simulink model "Simulink_Program"  (R2023b)
settings: Solver=VariableStepAuto  StartTime=0.0  StopTime=1  RelTol=1e-3
undefined symbols (not defined in the file or in its folder): battery_builder_rtmsupport, gcbh, Ns_Module, NumModules
libraries: nesl_utility x52, BatteryPack_105s34p_Library_lib x36, fl_lib x17, ee_lib x7
(part 1 of 5)
settings Model: Creator=romul  LastModifiedBy=OWNER

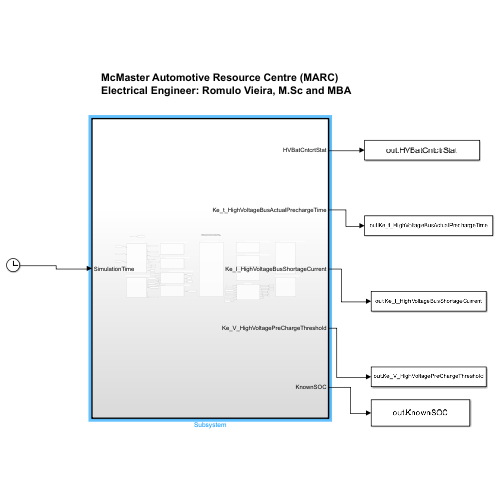
[thumbnail: Simulink's stored preview of the top-level diagram]
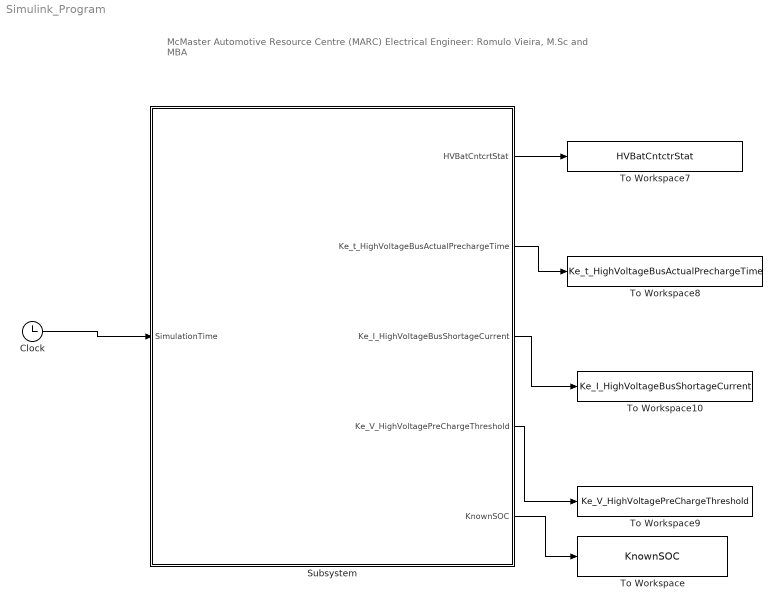
== system Simulink_Program ==
  note: McMaster Automotive Resource Centre (MARC)
      | Electrical Engineer: Romulo Vieira, M.Sc and MBA
  Clock : Clock
  Subsystem : Subsystem  TreatAsAtomicUnit=on
  To Workspace : ToWorkspace  VariableName=KnownSOC  SaveFormat=Timeseries  SampleTime=-1
  To Workspace10 : ToWorkspace  VariableName=Ke_I_HighVoltageBusShortageCurrent  SampleTime=-1
  To Workspace7 : ToWorkspace  VariableName=HVBatCntctrStat  SampleTime=-1
  To Workspace8 : ToWorkspace  VariableName=Ke_t_HighVoltageBusActualPrechargeTime  SampleTime=-1
  To Workspace9 : ToWorkspace  VariableName=Ke_V_HighVoltagePreChargeThreshold  SampleTime=-1
  wires:
  Subsystem/1(HVBatCntcrtStat) -> To Workspace7/1
  Subsystem/2(Ke_t_HighVoltageBusActualPrechargeTime) -> To Workspace8/1
  Subsystem/3(Ke_I_HighVoltageBusShortageCurrent) -> To Workspace10/1
  Clock/1 -> Subsystem/1(SimulationTime)
  Subsystem/4(Ke_V_HighVoltagePreChargeThreshold) -> To Workspace9/1
  Subsystem/5(KnownSOC) -> To Workspace/1

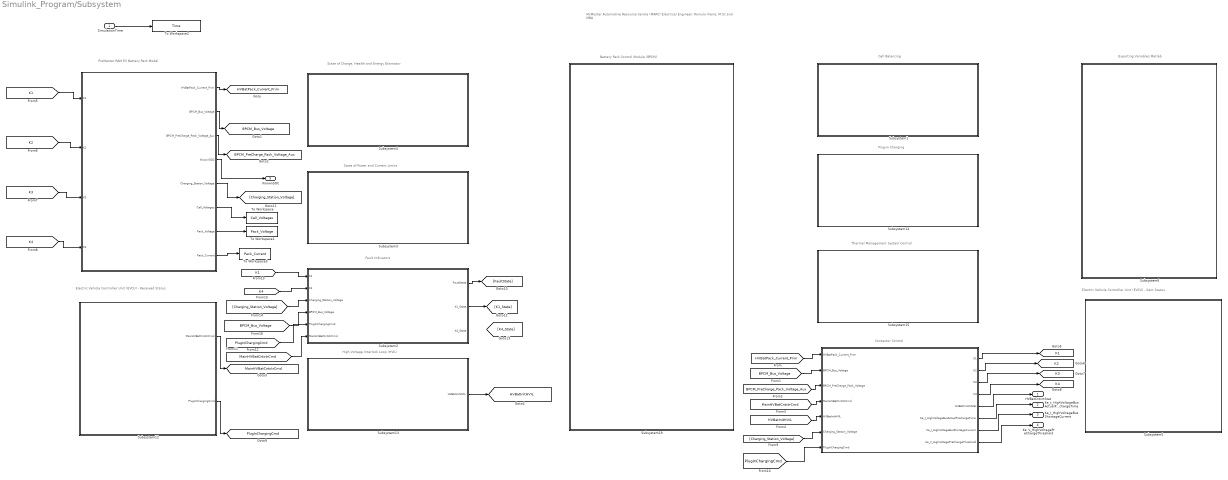
== system Simulink_Program/Subsystem ==
  note: McMaster Automotive Resource Centre (MARC)
      | Electrical Engineer: Romulo Vieira, M.Sc and MBA
  note: ProMaster RAM EV Battery Pack Model
  note: Contactor Control
  note: Battery Pack Control Module (BPCM)
  note: Thermal Management System Control
  note: Plug-In Charging
  note: Cell Balancing
  note: High Voltage Interlock Loop (HVIL)
  note: Fault Indicators
  note: State of Power and Current Limits
  note: State of Charge, Health and Energy Estimator
  note: Electric Vehicle Controller Unit (EVCU) - Received Status
  note: Electric Vehicle Controller Unit (EVCU) - Sent Status
  note: Exporting Variables Matlab
  SimulationTime : Inport
  " " : Subsystem  TreatAsAtomicUnit=on
  "  " : Subsystem  TreatAsAtomicUnit=on  SystemSampleTime=0.001
  Subsystem1 : Subsystem
  Subsystem12 : Subsystem
  Subsystem13 : Subsystem
  Subsystem14 : Subsystem
  Subsystem15 : Subsystem
  Subsystem19 : Subsystem
  Subsystem2 : Subsystem
  Subsystem3 : Subsystem
  Subsystem4 : Subsystem
  Subsystem5 : Subsystem
  Subsystem6 : Subsystem
  To Workspace : ToWorkspace  VariableName=Cell_Voltages  SaveFormat=Timeseries  SampleTime=-1
  To Workspace1 : ToWorkspace  VariableName=Pack_Voltage  SaveFormat=Timeseries  SampleTime=-1
  To Workspace2 : ToWorkspace  VariableName=Time  SampleTime=0.001
  To Workspace3 : ToWorkspace  VariableName=Pack_Current  SaveFormat=Timeseries  SampleTime=-1
  HVBatCntcrtStat : Outport
  Ke_t_HighVoltageBusActualPrechargeTime : Outport  Port=2
  Ke_I_HighVoltageBusShortageCurrent : Outport  Port=3
  Ke_V_HighVoltagePreChargeThreshold : Outport  Port=4
  KnownSOC : Outport  Port=5
  tag scope: BPCM_Bus_Voltage=global, BPCM_PreCharge_Pack_Voltage_Aux=global, HVBatInitHVIL=global, HVBatPack_Current_Prim=global, K1=global, K2=global, K3=global, K4=global, MainHVBatCntctrCmd=global, PlugInChargingCmd=global
  wires:
  "  "/5(HVBatCntctrStat) -> HVBatCntcrtStat/1
  "  "/6(Ke_t_HighVoltageBusActualPrechargeTime) -> Ke_t_HighVoltageBusActualPrechargeTime/1
  "  "/7(Ke_I_HighVoltageBusShortageCurrent) -> Ke_I_HighVoltageBusShortageCurrent/1
  "  "/8(Ke_V_HighVoltagePreChargeThreshold) -> Ke_V_HighVoltagePreChargeThreshold/1
  SimulationTime/1 -> To Workspace2/1
  " "/1(HVBatPack_Current_Prim) -> [HVBatPack_Current_Prim]
  " "/2(BPCM_Bus_Voltage) -> [BPCM_Bus_Voltage]
  " "/3(BPCM_PreCharge_Pack_Voltage_Aux) -> [BPCM_PreCharge_Pack_Voltage_Aux]
  [HVBatPack_Current_Prim] -> "  "/1(HVBatPack_Current_Prim)
  [BPCM_Bus_Voltage] -> "  "/2(BPCM_Bus_Voltage)
  [BPCM_PreCharge_Pack_Voltage_Aux] -> "  "/3(BPCM_PreCharge_Pack_Voltage)
  Subsystem12/1(" MainHVBatCntctrCmd      ") -> [MainHVBatCntctrCmd]
  [MainHVBatCntctrCmd] -> "  "/4(MainHVBatCntctrCmd)
  Subsystem13/1("HVBatInitHVIL   ") -> [HVBatInitHVIL]
  [HVBatInitHVIL] -> "  "/5(HVBatInitHVIL)
  "  "/3(K3) -> [K3]
  "  "/4(K4) -> [K4]
  "  "/1(K1) -> [K1]
  "  "/2(K2) -> [K2]
  [K1] -> " "/1(K1)
  [K2] -> " "/2(K2)
  [K3] -> " "/3(K3)
  [K4] -> " "/4(K4)
  " "/4(KnownSOC) -> KnownSOC/1
  " "/5(Charging_Station_Voltage) -> [Charging_Station_Voltage]
  [Charging_Station_Voltage] -> "  "/6(Charging_Station_Voltage)
  " "/6(Cell_Voltages) -> To Workspace/1
  " "/7(Pack_Voltage) -> To Workspace1/1
  " "/8(Pack_Current) -> To Workspace3/1
  [PlugInChargingCmd] -> "  "/7(PlugInChargingCmd)
  Subsystem12/2(" PlugInChargingCmd      ") -> [PlugInChargingCmd]
  [K1] -> Subsystem2/1(K1)
  [BPCM_Bus_Voltage] -> Subsystem2/4(BPCM_Bus_Voltage)
  [K4] -> Subsystem2/2(K4)
  [Charging_Station_Voltage] -> Subsystem2/3(Charging_Station_Voltage)
  [PlugInChargingCmd] -> Subsystem2/5(PlugInChargingCmd)
  [MainHVBatCntctrCmd] -> Subsystem2/6(MainHVBatCntctrCmd)
  Subsystem2/1(FaultState) -> [FaultState]
  Subsystem2/2(K1_State) -> [K1_State]

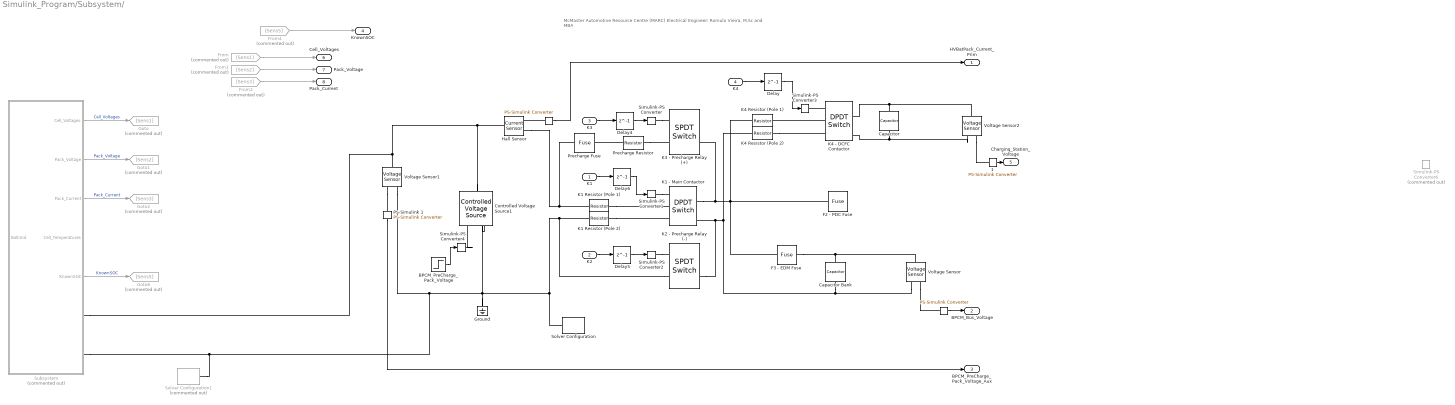
== system Simulink_Program/Subsystem/  ==
  note: McMaster Automotive Resource Centre (MARC)
      | Electrical Engineer: Romulo Vieira, M.Sc and MBA
  K1 : Inport
  K2 : Inport  Port=2
  K3 : Inport  Port=3
  K4 : Inport  Port=4
  "   " : nesl_utility/PS-Simulink Converter  PhysicalDomain=network_engine_domain  SubClassName=ps_output  LeftPortType=input  RightPortType=output  PseudoPeriodic=off  Frequencies=[]  VectorFormat=inherit  Unit=inherit  AffineConversion=off
  " " : nesl_utility/PS-Simulink Converter  PhysicalDomain=network_engine_domain  SubClassName=ps_output  LeftPortType=input  RightPortType=output  PseudoPeriodic=off  Frequencies=[]  VectorFormat=inherit  Unit=inherit  AffineConversion=off
  " 1" : nesl_utility/PS-Simulink Converter  PhysicalDomain=network_engine_domain  SubClassName=ps_output  LeftPortType=input  RightPortType=output  PseudoPeriodic=off  Frequencies=[]  VectorFormat=inherit  Unit=inherit  AffineConversion=off
  BPCM_PreCharge_Pack_Voltage : Step  Time=0  After=450  SampleTime=0.001
  Capacitor : fl_lib/Electrical/Electrical Elements/Capacitor  c=750e-6 F  r=1e-6 Ohm  g=0 1/Ohm  i_specify=off  i_priority=None  i=0 A  i_nominal_specify=off  i_nominal_unit=A  i_nominal_value=1  v_specify=off  v_priority=None  v=0 V  v_nominal_specify=off  v_nominal_unit=V  v_nominal_value=1  vc_specify=off  vc_priority=High  vc=0 V  vc_nominal_specify=off  vc_nominal_unit=V  vc_nominal_value=1
  Capacitor Bank : fl_lib/Electrical/Electrical Elements/Capacitor  c=750e-6 F  r=1e-6 Ohm  g=0 1/Ohm  i_specify=off  i_priority=None  i=0 A  i_nominal_specify=off  i_nominal_unit=A  i_nominal_value=1  v_specify=off  v_priority=None  v=0 V  v_nominal_specify=off  v_nominal_unit=V  v_nominal_value=1  vc_specify=on  vc_priority=High  vc=0 V  vc_nominal_specify=off  vc_nominal_unit=V  vc_nominal_value=1
  Controlled Voltage Source1 : fl_lib/Electrical/Electrical Sources/Controlled Voltage Source
  Delay{,4..6} (4 alike) : Delay  DelayLength=1
  F2 - PDC Fuse : ee_lib/Switches & Breakers/Fuse  prm=1  I_rated=125 A  melt_margin=1  T_fuse=0 s  I2t=1 A^2*s  I_vec=[1.9, 2, 2.5, 30] A  t_vec=[10000, 1, .3, .001] s  R_closed=0.01 Ohm  G_open=1e-8 1/Ohm  exposemeasurement=ee.enum.exposemeasurement.hidden
      settings: InternalSimscapePortConfiguration="{\"Bottom\":[],\"Left\":[{\"id\":\"p\",\"label\":\"\",\"type\":\"foundation.electrical.electrical\"}],\"Right\":[{\"id\":\"n\",\"label\":\"\",\"type\":\"foundation.electrical.electrical\"}],\"Top\":[]}"
  F3 - EDM Fuse : ee_lib/Switches & Breakers/Fuse  prm=1  I_rated=600 A  melt_margin=1  T_fuse=0 s  I2t=1 A^2*s  I_vec=[1.9, 2, 2.5, 30] A  t_vec=[10000, 1, .3, .001] s  R_closed=0.01 Ohm  G_open=1e-8 1/Ohm  exposemeasurement=ee.enum.exposemeasurement.hidden
      settings: InternalSimscapePortConfiguration="{\"Bottom\":[],\"Left\":[{\"id\":\"p\",\"label\":\"\",\"type\":\"foundation.electrical.electrical\"}],\"Right\":[{\"id\":\"n\",\"label\":\"\",\"type\":\"foundation.electrical.electrical\"}],\"Top\":[]}"
  From : From  Commented=on  GotoTag=Sens1
  From1 : From  Commented=on  GotoTag=Sens2
  From2 : From  Commented=on  GotoTag=Sens3
  From4 : From  Commented=on  GotoTag=Sens5
  Goto : Goto  Commented=on  GotoTag=Sens1
  Goto1 : Goto  Commented=on  GotoTag=Sens2
  Goto2 : Goto  Commented=on  GotoTag=Sens3
  Goto6 : Goto  Commented=on  GotoTag=Sens5
  Ground : fl_lib/Electrical/Electrical Elements/Electrical Reference
  Hall Sensor : fl_lib/Electrical/Electrical Sensors/Current Sensor
  K1 - Main Contactor : ee_lib/Switches & Breakers/DPDT Switch  R_closed=0.01 Ohm  G_open=1e-6 S  Threshold=0.5 V  Width=0 V  model_dynamics=0  t_on=1e-3 s  t_off=1e-3 s  initial_vT=0 V
      settings: InternalSimscapePortConfiguration="{\"Bottom\":[],\"Left\":[{\"id\":\"vT\",\"label\":\"vT\",\"type\":\"input\"},{\"id\":\"p1\",\"label\":\"\",\"type\":\"foundation.electrical.electrical\"},{\"id\":\"p2\",\"label\":\"\",\"type\":\"foundation.electrical.electrical\"}],\"Right\":[{\"id\":\"n11\",\"label\":\"\",\"type\":\"foundation.electrical.electrical\"},{\"id\":\"n12\",\"label\":\"\",\"type\":\"foundation.electrical.electrical\"},{\"id\":\"n21\",\"label\":\"\",\"type\":\"foundation.electrical.electrical\"},{\"id\":\"n22\",\"label\":\"\",\"type\":\"foundation.electrical.electrical\"}],\"Top\":[]}"
  K1 Resistor (Pole 1) : fl_lib/Electrical/Electrical Elements/Resistor  R=0.0003 Ohm  i_specify=off  i_priority=None  i=0 A  i_nominal_specify=off  i_nominal_unit=A  i_nominal_value=1  v_specify=off  v_priority=None  v=0 V  v_nominal_specify=off  v_nominal_unit=V  v_nominal_value=1
  K1 Resistor (Pole 2) : fl_lib/Electrical/Electrical Elements/Resistor  R=0.0003 Ohm  i_specify=off  i_priority=None  i=0 A  i_nominal_specify=off  i_nominal_unit=A  i_nominal_value=1  v_specify=off  v_priority=None  v=0 V  v_nominal_specify=off  v_nominal_unit=V  v_nominal_value=1
  K2 - Precharge Relay (-) : ee_lib/Switches & Breakers/SPDT Switch  R_closed=0.01 Ohm  G_open=1e-6 S  Threshold=0.5 V  Width=0 V  model_dynamics=0  t_on=1e-3 s  t_off=1e-3 s  initial_vT=0 V
  K3 - Precharge Relay (+) : ee_lib/Switches & Breakers/SPDT Switch  R_closed=0.01 Ohm  G_open=1e-6 S  Threshold=0.5 V  Width=0 V  model_dynamics=0  t_on=1e-3 s  t_off=1e-3 s  initial_vT=0 V
  K4 - DCFC Contactor : ee_lib/Switches & Breakers/DPDT Switch  R_closed=0.01 Ohm  G_open=1e-6 S  Threshold=0.5 V  Width=0 V  model_dynamics=0  t_on=1e-3 s  t_off=1e-3 s  initial_vT=0 V
      settings: InternalSimscapePortConfiguration="{\"Bottom\":[],\"Left\":[{\"id\":\"vT\",\"label\":\"vT\",\"type\":\"input\"},{\"id\":\"p1\",\"label\":\"\",\"type\":\"foundation.electrical.electrical\"},{\"id\":\"p2\",\"label\":\"\",\"type\":\"foundation.electrical.electrical\"}],\"Right\":[{\"id\":\"n11\",\"label\":\"\",\"type\":\"foundation.electrical.electrical\"},{\"id\":\"n12\",\"label\":\"\",\"type\":\"foundation.electrical.electrical\"},{\"id\":\"n21\",\"label\":\"\",\"type\":\"foundation.electrical.electrical\"},{\"id\":\"n22\",\"label\":\"\",\"type\":\"foundation.electrical.electrical\"}],\"Top\":[]}"
  K4 Resistor (Pole 1) : fl_lib/Electrical/Electrical Elements/Resistor  R=0.0003 Ohm  i_specify=off  i_priority=None  i=0 A  i_nominal_specify=off  i_nominal_unit=A  i_nominal_value=1  v_specify=off  v_priority=None  v=0 V  v_nominal_specify=off  v_nominal_unit=V  v_nominal_value=1
  K4 Resistor (Pole 2) : fl_lib/Electrical/Electrical Elements/Resistor  R=0.0003 Ohm  i_specify=off  i_priority=None  i=0 A  i_nominal_specify=off  i_nominal_unit=A  i_nominal_value=1  v_specify=off  v_priority=None  v=0 V  v_nominal_specify=off  v_nominal_unit=V  v_nominal_value=1
  PS-Simulink 1 : nesl_utility/PS-Simulink Converter  PhysicalDomain=network_engine_domain  SubClassName=ps_output  LeftPortType=input  RightPortType=output  PseudoPeriodic=off  Frequencies=[]  VectorFormat=inherit  Unit=inherit  AffineConversion=off
  Precharge Fuse : ee_lib/Switches & Breakers/Fuse  prm=1  I_rated=600 A  melt_margin=1  T_fuse=0 s  I2t=1 A^2*s  I_vec=[1.9, 2, 2.5, 30] A  t_vec=[10000, 1, .3, .001] s  R_closed=0.01 Ohm  G_open=1e-8 1/Ohm  exposemeasurement=ee.enum.exposemeasurement.hidden
      settings: InternalSimscapePortConfiguration="{\"Bottom\":[],\"Left\":[{\"id\":\"p\",\"label\":\"\",\"type\":\"foundation.electrical.electrical\"}],\"Right\":[{\"id\":\"n\",\"label\":\"\",\"type\":\"foundation.electrical.electrical\"}],\"Top\":[]}"
  Precharge Resistor : fl_lib/Electrical/Electrical Elements/Resistor  R=25 Ohm  i_specify=off  i_priority=None  i=0 A  i_nominal_specify=off  i_nominal_unit=A  i_nominal_value=1  v_specify=off  v_priority=None  v=0 V  v_nominal_specify=off  v_nominal_unit=V  v_nominal_value=1
  Simulink-PS Converter{,1..3} (4 alike) : nesl_utility/Simulink-PS Converter  PhysicalDomain=network_engine_domain  SubClassName=ps_input  LeftPortType=input  RightPortType=output  PseudoPeriodic=off  Frequencies=[]  NoiseDistribution=none  NoiseParameters=[]  Unit=1  AffineConversion=off  FilteringAndDerivatives=provide  SimscapeFilterOrder=1  InputFilterTimeConstant=0.001  UdotUserProvided=0
  Simulink-PS Converter4 : nesl_utility/Simulink-PS Converter  PhysicalDomain=network_engine_domain  SubClassName=ps_input  LeftPortType=input  RightPortType=output  PseudoPeriodic=off  Frequencies=[]  NoiseDistribution=none  NoiseParameters=[]  Unit=1  AffineConversion=off  FilteringAndDerivatives=filter  SimscapeFilterOrder=1  InputFilterTimeConstant=0.0000001  UdotUserProvided=0
  Simulink-PS Converter6 : nesl_utility/Simulink-PS Converter  Commented=on  PhysicalDomain=network_engine_domain  SubClassName=ps_input  LeftPortType=input  RightPortType=output  PseudoPeriodic=off  Frequencies=[]  NoiseDistribution=none  NoiseParameters=[]  Unit=1  AffineConversion=off  FilteringAndDerivatives=provide  SimscapeFilterOrder=1  InputFilterTimeConstant=0.001  UdotUserProvided=0
  Solver Configuration : nesl_utility/Solver Configuration  PhysicalDomain=network_engine_domain  SubClassName=solver  LeftPortType=input  RightPortType=generic  Tones=[]  Harmonics=[]  SimulateNoise=off  Profile=off  UseLocalSampling=off  EnableSwitchedLinearOptims=on  FrequencyDomain=off  UseCCode=off  RelTol=0.001  AbsTol=0.001  MinStep=1e-09  ToWorkspace=off  RevertToSquareIcSolve=off  NumHomotopyIterations=100  PhasorMode=off  PhasorModeNumHarmonics=1  ConsistencySolver=NEWTON_XTOL_AFTER_FTOL  IndexReductionMethod=DerivativeReplacement  DoDC=off  ResidualTolerance=1e-09  ConsistencyTolSource=GLOBAL  ConsistencyAbsTol=0.001  ConsistencyRelTol=0.001  ConsistencyTolFactor=0.001  UseLocalSolver=on  LocalSolverChoice=NE_BACKWARD_EULER_ADVANCER  ResolveIndetEquations=on  FunctionEvalNumThread=1  LocalSolverSampleTime=0.001  DoFixedCost=on  MaxNonlinIter=3  MaxModeIter=2  ComputeImpulses=off  ImpulseIterations=2  LinearAlgebra=auto  LinearAlgebraNumThread=0  EquationFormulation=NE_TIME_EF  DelaysMemoryBudget=1024  AutomaticFiltering=off  FilteringTimeConstant=0.001  PartitionStorageMethod=AS_NEEDED  PartitionMemoryBudget=1024  PartitionMethod=ROBUST  MultibodyUseLocalSolver=off  MultibodyLocalSolverChoice=ODE1  MultibodyLocalSolverSampleTime=0.001
  Solver Configuration1 : nesl_utility/Solver Configuration  Commented=on  PhysicalDomain=network_engine_domain  SubClassName=solver  LeftPortType=input  RightPortType=generic  Tones=[]  Harmonics=[]  SimulateNoise=off  Profile=off  UseLocalSampling=off  EnableSwitchedLinearOptims=on  FrequencyDomain=off  UseCCode=off  RelTol=0.001  AbsTol=0.001  MinStep=1e-09  ToWorkspace=off  RevertToSquareIcSolve=off  NumHomotopyIterations=100  PhasorMode=off  PhasorModeNumHarmonics=1  ConsistencySolver=NEWTON_XTOL_AFTER_FTOL  IndexReductionMethod=DerivativeReplacement  DoDC=off  ResidualTolerance=1e-09  ConsistencyTolSource=GLOBAL  ConsistencyAbsTol=0.001  ConsistencyRelTol=0.001  ConsistencyTolFactor=0.001  UseLocalSolver=on  LocalSolverChoice=NE_BACKWARD_EULER_ADVANCER  ResolveIndetEquations=on  FunctionEvalNumThread=1  LocalSolverSampleTime=0.001  DoFixedCost=on  MaxNonlinIter=3  MaxModeIter=2  ComputeImpulses=off  ImpulseIterations=2  LinearAlgebra=auto  LinearAlgebraNumThread=0  EquationFormulation=NE_TIME_EF  DelaysMemoryBudget=1024  AutomaticFiltering=off  FilteringTimeConstant=0.001  PartitionStorageMethod=AS_NEEDED  PartitionMemoryBudget=1024  PartitionMethod=ROBUST  MultibodyUseLocalSolver=off  MultibodyLocalSolverChoice=ODE1  MultibodyLocalSolverSampleTime=0.001
  Subsystem : Subsystem  Commented=on
      mask Display: image('saft-stellantis.jpg', [20, 45, 120, 70]);
  Voltage Sensor : fl_lib/Electrical/Electrical Sensors/Voltage Sensor
  Voltage Sensor1 : fl_lib/Electrical/Electrical Sensors/Voltage Sensor
  Voltage Sensor2 : fl_lib/Electrical/Electrical Sensors/Voltage Sensor
  HVBatPack_Current_Prim : Outport
  BPCM_Bus_Voltage : Outport  Port=2
  BPCM_PreCharge_Pack_Voltage_Aux : Outport  Port=3
  KnownSOC : Outport  Port=4  VectorParamsAs1DForOutWhenUnconnected=off  BusOutputAsStruct=on
  Charging_Station_Voltage : Outport  Port=5
  Cell_Voltages : Outport  Port=6
  Pack_Voltage : Outport  Port=7
  Pack_Current : Outport  Port=8
  wires:
  "   "/1 -> HVBatPack_Current_Prim/1
  K1/1 -> Delay6/1
  K2/1 -> Delay5/1
  BPCM_PreCharge_Pack_Voltage/1 -> Simulink-PS Converter4/1
  K3/1 -> Delay4/1
  Delay4/1 -> Simulink-PS Converter/1
  K4/1 -> Delay/1
  Delay5/1 -> Simulink-PS Converter2/1
  PS-Simulink 1/1 -> BPCM_PreCharge_Pack_Voltage_Aux/1
  " "/1 -> BPCM_Bus_Voltage/1
  Subsystem/1(Cell_Voltages) -> Goto/1  "Cell_Voltages"
  Subsystem/5(KnownSOC) -> Goto6/1  "KnownSOC"
  Subsystem/3(Pack_Current) -> Goto2/1  "Pack_Current"
  Subsystem/2(Pack_Voltage) -> Goto1/1  "Pack_Voltage"
  From1/1 -> Pack_Voltage/1
  From/1 -> Cell_Voltages/1
  From4/1 -> KnownSOC/1
  From2/1 -> Pack_Current/1
  " 1"/1 -> Charging_Station_Voltage/1
  Delay6/1 -> Simulink-PS Converter1/1
  Delay/1 -> Simulink-PS Converter3/1
  connections:
  K1 Resistor (Pole 2)/LConn1 -- K1 - Main Contactor/LConn3
  Capacitor Bank/LConn1 -- Voltage Sensor/LConn1 -- F3 - EDM Fuse/LConn1
  K2 - Precharge Relay (-)/RConn2 -- K1 - Main Contactor/RConn4 -- Voltage Sensor/RConn2 -- Capacitor Bank/RConn1 -- K4 Resistor (Pole 2)/RConn1
  Hall Sensor/RConn2 -- Precharge Fuse/LConn1 -- K1 Resistor (Pole 1)/RConn1
  K3 - Precharge Relay (+)/RConn2 -- K4 Resistor (Pole 1)/RConn1 -- F2 - PDC Fuse/RConn1 -- F3 - EDM Fuse/RConn1 -- K1 - Main Contactor/RConn2
  Precharge Resistor/LConn1 -- K3 - Precharge Relay (+)/LConn2
  Simulink-PS Converter2/RConn1 -- K2 - Precharge Relay (-)/LConn1
  Precharge Resistor/RConn1 -- Precharge Fuse/RConn1
  Simulink-PS Converter1/RConn1 -- K1 - Main Contactor/LConn1
  Controlled Voltage Source1/LConn1 -- Subsystem/RConn1 -- Voltage Sensor1/LConn1 -- Hall Sensor/LConn1
  Simulink-PS Converter/RConn1 -- K3 - Precharge Relay (+)/LConn1
  Voltage Sensor/RConn1 -- " "/LConn1
  K4 - DCFC Contactor/LConn1 -- Simulink-PS Converter3/RConn1
  "   "/LConn1 -- Hall Sensor/RConn1
  Simulink-PS Converter4/RConn1 -- Controlled Voltage Source1/RConn1
  Voltage Sensor1/RConn1 -- PS-Simulink 1/LConn1
  K1 Resistor (Pole 1)/LConn1 -- K1 - Main Contactor/LConn2
  Solver Configuration/RConn1 -- Solver Configuration1/RConn1 -- Subsystem/RConn2 -- Voltage Sensor1/RConn2 -- Ground/LConn1 -- Controlled Voltage Source1/RConn2 -- K2 - Precharge Relay (-)/LConn2 -- K1 Resistor (Pole 2)/RConn1
  K4 - DCFC Contactor/LConn2 -- K4 Resistor (Pole 1)/LConn1
  K4 Resistor (Pole 2)/LConn1 -- K4 - DCFC Contactor/LConn3
  Voltage Sensor2/LConn1 -- Capacitor/LConn1 -- K4 - DCFC Contactor/RConn2
  Voltage Sensor2/RConn2 -- K4 - DCFC Contactor/RConn4 -- Capacitor/RConn1
  Voltage Sensor2/RConn1 -- " 1"/LConn1

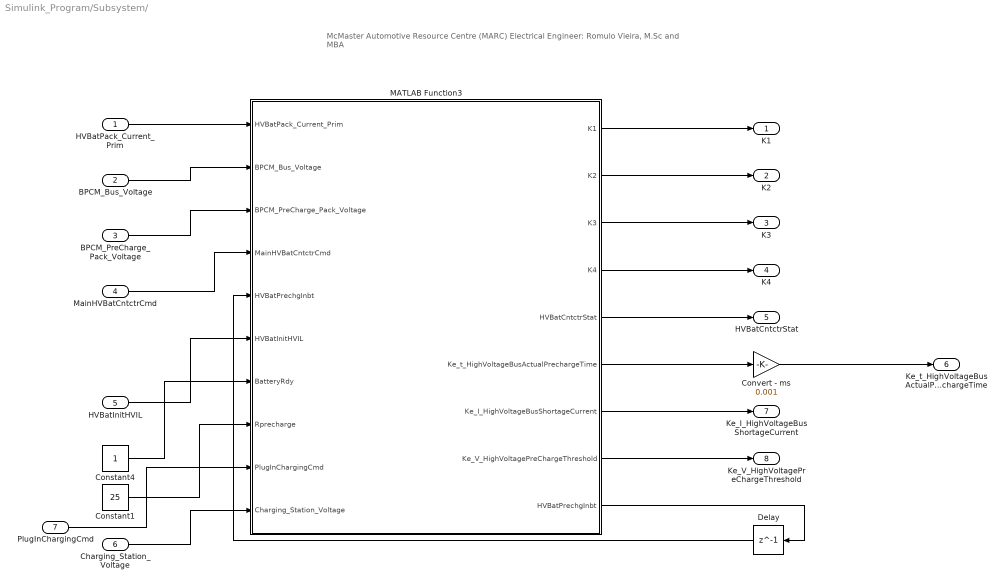
== system Simulink_Program/Subsystem/   ==
  note: McMaster Automotive Resource Centre (MARC)
      | Electrical Engineer: Romulo Vieira, M.Sc and MBA
  HVBatPack_Current_Prim : Inport
  BPCM_Bus_Voltage : Inport  Port=2
  BPCM_PreCharge_Pack_Voltage : Inport  Port=3
  MainHVBatCntctrCmd : Inport  Port=4
  HVBatInitHVIL : Inport  Port=5
  Charging_Station_Voltage : Inport  Port=6
  PlugInChargingCmd : Inport  Port=7
  Constant1 : Constant  Value=25
  Constant4 : Constant
  Convert - ms : Gain  Gain=0.001
  Delay : Delay  DelayLength=1
  MATLAB Function3 : MATLAB Function  SystemSampleTime=0.001
  K1 : Outport
  K2 : Outport  Port=2
  K3 : Outport  Port=3
  K4 : Outport  Port=4
  HVBatCntctrStat : Outport  Port=5
  Ke_t_HighVoltageBusActualPrechargeTime : Outport  Port=6
  Ke_I_HighVoltageBusShortageCurrent : Outport  Port=7
  Ke_V_HighVoltagePreChargeThreshold : Outport  Port=8
  wires:
  Constant4/1 -> MATLAB Function3/7(BatteryRdy)
  HVBatPack_Current_Prim/1 -> MATLAB Function3/1(HVBatPack_Current_Prim)
  BPCM_PreCharge_Pack_Voltage/1 -> MATLAB Function3/3(BPCM_PreCharge_Pack_Voltage)
  HVBatInitHVIL/1 -> MATLAB Function3/6(HVBatInitHVIL)
  MATLAB Function3/4(K4) -> K4/1
  BPCM_Bus_Voltage/1 -> MATLAB Function3/2(BPCM_Bus_Voltage)
  MainHVBatCntctrCmd/1 -> MATLAB Function3/4(MainHVBatCntctrCmd)
  MATLAB Function3/1(K1) -> K1/1
  Constant1/1 -> MATLAB Function3/8(Rprecharge)
  MATLAB Function3/2(K2) -> K2/1
  MATLAB Function3/3(K3) -> K3/1
  MATLAB Function3/5(HVBatCntctrStat) -> HVBatCntctrStat/1
  MATLAB Function3/6(Ke_t_HighVoltageBusActualPrechargeTime) -> Convert - ms/1
  MATLAB Function3/7(Ke_I_HighVoltageBusShortageCurrent) -> Ke_I_HighVoltageBusShortageCurrent/1
  MATLAB Function3/8(Ke_V_HighVoltagePreChargeThreshold) -> Ke_V_HighVoltagePreChargeThreshold/1
  Delay/1 -> MATLAB Function3/5("HVBatPrechgInbt ")
  MATLAB Function3/9(HVBatPrechgInbt) -> Delay/1
  Convert - ms/1 -> Ke_t_HighVoltageBusActualPrechargeTime/1
  Charging_Station_Voltage/1 -> MATLAB Function3/10(Charging_Station_Voltage)
  PlugInChargingCmd/1 -> MATLAB Function3/9(PlugInChargingCmd)

== system Simulink_Program/Subsystem/Subsystem1 ==

== system Simulink_Program/Subsystem/Subsystem12 ==
  note: McMaster Automotive Resource Centre (MARC)
      | Electrical Engineer: Romulo Vieira, M.Sc and MBA
  MainHVBatCntctrCmd : Step  Time=0.1  SampleTime=0.001
  PlugInChargingCmd : Step  Time=0.1  SampleTime=0.001
  " MainHVBatCntctrCmd      " : Outport
  " PlugInChargingCmd      " : Outport  Port=2
  wires:
  PlugInChargingCmd/1 -> " PlugInChargingCmd      "/1
  MainHVBatCntctrCmd/1 -> " MainHVBatCntctrCmd      "/1

== system Simulink_Program/Subsystem/Subsystem13 ==
  note: McMaster Automotive Resource Centre (MARC)
      | Electrical Engineer: Romulo Vieira, M.Sc and MBA
  HVBatInitHVIL : Constant
  "HVBatInitHVIL   " : Outport
  wires:
  HVBatInitHVIL/1 -> "HVBatInitHVIL   "/1

== system Simulink_Program/Subsystem/Subsystem14 ==

== system Simulink_Program/Subsystem/Subsystem15 ==

== system Simulink_Program/Subsystem/Subsystem19 ==

== system Simulink_Program/Subsystem/Subsystem2 ==
  K1 : Inport
  K4 : Inport  Port=2
  Charging_Station_Voltage : Inport  Port=3
  BPCM_Bus_Voltage : Inport  Port=4
  PlugInChargingCmd : Inport  Port=5
  MainHVBatCntctrCmd : Inport  Port=6
  MATLAB Function : MATLAB Function  TreatAsAtomicUnit=on
  FaultState : Outport
  K1_State : Outport  Port=2
  K4_State : Outport  Port=3
  wires:
  MainHVBatCntctrCmd/1 -> MATLAB Function/6(MainHVBatCntctrCmd)
  PlugInChargingCmd/1 -> MATLAB Function/5(PlugInChargingCmd)
  K1/1 -> MATLAB Function/1(K1)
  K4/1 -> MATLAB Function/2(K4)
  Charging_Station_Voltage/1 -> MATLAB Function/3(Charging_Station_Voltage)
  BPCM_Bus_Voltage/1 -> MATLAB Function/4(BPCM_Bus_Voltage)
  MATLAB Function/1(FaultState) -> FaultState/1
  MATLAB Function/2(K1_State) -> K1_State/1
  MATLAB Function/3(K4_State) -> K4_State/1

== system Simulink_Program/Subsystem/Subsystem3 ==

== system Simulink_Program/Subsystem/Subsystem4 ==

== system Simulink_Program/Subsystem/Subsystem5 ==

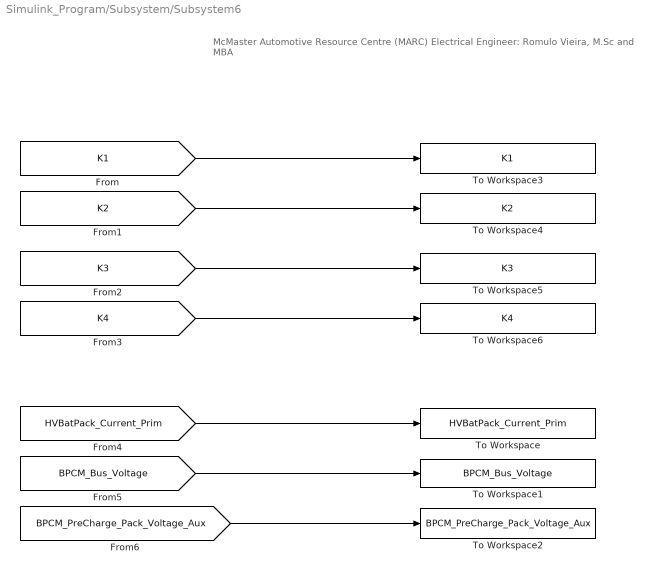
== system Simulink_Program/Subsystem/Subsystem6 ==
  note: McMaster Automotive Resource Centre (MARC)
      | Electrical Engineer: Romulo Vieira, M.Sc and MBA
  To Workspace : ToWorkspace  VariableName=HVBatPack_Current_Prim  SampleTime=-1
  To Workspace1 : ToWorkspace  VariableName=BPCM_Bus_Voltage  SampleTime=-1
  To Workspace2 : ToWorkspace  VariableName=BPCM_PreCharge_Pack_Voltage_Aux  SampleTime=-1
  To Workspace3 : ToWorkspace  VariableName=K1  SampleTime=-1
  To Workspace4 : ToWorkspace  VariableName=K2  SampleTime=-1
  To Workspace5 : ToWorkspace  VariableName=K3  SampleTime=-1
  To Workspace6 : ToWorkspace  VariableName=K4  SampleTime=-1
  wires:
  [K2] -> To Workspace4/1
  [K1] -> To Workspace3/1
  [K3] -> To Workspace5/1
  [K4] -> To Workspace6/1
  [HVBatPack_Current_Prim] -> To Workspace/1
  [BPCM_Bus_Voltage] -> To Workspace1/1
  [BPCM_PreCharge_Pack_Voltage_Aux] -> To Workspace2/1

== system Simulink_Program/Subsystem/ /Subsystem ==
  BalCmd : Inport
  BatteryPack_1Module : Subsystem  VariantControl=NumModules == 1
  BatteryPack_35Modules : Subsystem  VariantControl=NumModules == 16
  +Batt : PMIOPort  Side=Right
  -Batt : PMIOPort  Port=2  Side=Right
  Cell_Voltages : Outport  VectorParamsAs1DForOutWhenUnconnected=off
  Pack_Voltage : Outport  Port=2  VectorParamsAs1DForOutWhenUnconnected=off
  Pack_Current : Outport  Port=3  VectorParamsAs1DForOutWhenUnconnected=off
  Cell_Temperatures : Outport  Port=4  VectorParamsAs1DForOutWhenUnconnected=off
  KnownSOC : Outport  Port=5  VectorParamsAs1DForOutWhenUnconnected=off

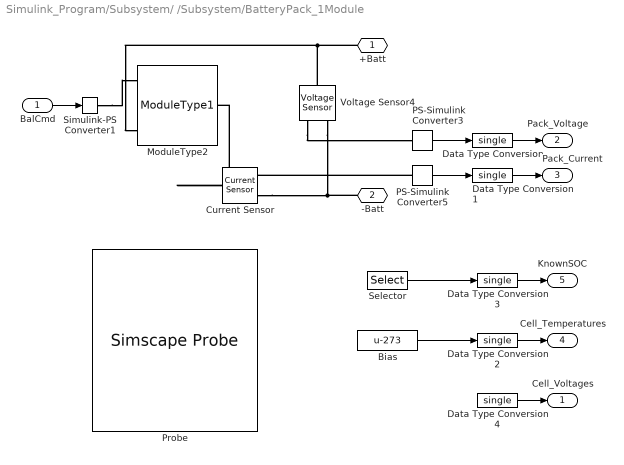
== system Simulink_Program/Subsystem/ /Subsystem/BatteryPack_1Module ==
  BalCmd : Inport
  Bias : Bias  Bias=-273  SaturateOnIntegerOverflow=off
  Current Sensor : fl_lib/Electrical/Electrical Sensors/Current Sensor
  Data Type Conversion{,1..4} (5 alike) : DataTypeConversion  OutDataTypeStr=single  SaturateOnIntegerOverflow=off  RndMeth=Floor
  ModuleType2 : BatteryPack_105s34p_Library_lib/Modules/ModuleType1  SOC_vecCell=ModuleType1.SOC_vecCell  T_vecCell=ModuleType1.T_vecCell K  V0_matCell=ModuleType1.V0_matCell V  V_rangeCell=ModuleType1.V_rangeCell V  R0_matCell=ModuleType1.R0_matCell Ohm  AHCell=ModuleType1.AHCell A*hr  extrapolation_optionCell=simscape.enum.extrapolation.nearest  thermal_massCell=ModuleType1.thermal_massCell J/K  CoolantResistance=ModuleType1.CoolantResistance K/W  CellBalancingClosedResistance=ModuleType1.CellBalancingClosedResistance Ohm  CellBalancingOpenConductance=ModuleType1.CellBalancingOpenConductance 1/Ohm  CellBalancingThreshold=ModuleType1.CellBalancingThreshold  CellBalancingResistance=ModuleType1.CellBalancingResistance Ohm  P=34  S=3  iCell_specify=off  iCell_priority=None  iCell=repmat(0, 102, 1) A  iCell_nominal_specify=off  iCell_nominal_unit=A  iCell_nominal_value=1  vCell_specify=off  vCell_priority=None  vCell=repmat(0, 102, 1) V  vCell_nominal_specify=off  vCell_nominal_unit=V  vCell_nominal_value=1  socCell_specify=off  socCell_priority=High  socCell=repmat(1, 102, 1)  socCell_nominal_specify=off  socCell_nominal_unit=1  socCell_nominal_value=1  numCyclesCell_specify=off  numCyclesCell_priority=High  numCyclesCell=repmat(0, 102, 1)  numCyclesCell_nominal_specify=off  numCyclesCell_nominal_unit=1  numCyclesCell_nominal_value=1  temperatureCell_specify=off  temperatureCell_priority=High  temperatureCell=repmat(298.15, 102, 1) K  temperatureCell_nominal_specify=off  temperatureCell_nominal_unit=K  temperatureCell_nominal_value=1  vParallelAssembly_specify=off  vParallelAssembly_priority=None  vParallelAssembly=repmat(0, 3, 1) V  vParallelAssembly_nominal_specify=off  vParallelAssembly_nominal_unit=V  vParallelAssembly_nominal_value=1  socParallelAssembly_specify=off  socParallelAssembly_priority=None  socParallelAssembly=repmat(1, 3, 1)  socParallelAssembly_nominal_specify=off  socParallelAssembly_nominal_unit=1  socParallelAssembly_nominal_value=1
      settings: InternalSimscapePortConfiguration="{\"Bottom\":[{\"id\":\"n\",\"label\":\"-\",\"type\":\"foundation.electrical.electrical\"}],\"Left\":[{\"id\":\"enableCellBalancing\",\"label\":\"CB\",\"type\":\"input\"},{\"id\":\"ClntH\",\"label\":\"ClntH\",\"type\":\"foundation.thermal.thermal\"}],\"Right\":[],\"Top\":[{\"id\":\"p\",\"label\":\"+\",\"type\":\"foundation.electrical.electrical\"}]}"
  PS-Simulink Converter3 : nesl_utility/PS-Simulink Converter  PhysicalDomain=network_engine_domain  SubClassName=ps_output  LeftPortType=input  RightPortType=output  PseudoPeriodic=off  Frequencies=[]  VectorFormat=1-D array  Unit=V  AffineConversion=off
  PS-Simulink Converter5 : nesl_utility/PS-Simulink Converter  PhysicalDomain=network_engine_domain  SubClassName=ps_output  LeftPortType=input  RightPortType=output  PseudoPeriodic=off  Frequencies=[]  VectorFormat=1-D array  Unit=A  AffineConversion=off
  Probe : SimscapeProbe
  Selector : Selector  InputPortWidth=NumModules*Ns_Module  IndexOptions=Index vector (dialog)  Indices=1  OutputSizes=1
  Simulink-PS Converter1 : nesl_utility/Simulink-PS Converter  PhysicalDomain=network_engine_domain  SubClassName=ps_input  LeftPortType=input  RightPortType=output  PseudoPeriodic=off  Frequencies=[]  NoiseDistribution=none  NoiseParameters=[]  Unit=1  AffineConversion=off  FilteringAndDerivatives=provide  SimscapeFilterOrder=1  InputFilterTimeConstant=0.001  UdotUserProvided=0
  Voltage Sensor4 : fl_lib/Electrical/Electrical Sensors/Voltage Sensor
  +Batt : PMIOPort  Side=Right
  -Batt : PMIOPort  Port=2  Side=Right
  Cell_Voltages : Outport  VectorParamsAs1DForOutWhenUnconnected=off
  Pack_Voltage : Outport  Port=2  Unit=V  VectorParamsAs1DForOutWhenUnconnected=off
  Pack_Current : Outport  Port=3  Unit=A  VectorParamsAs1DForOutWhenUnconnected=off
  Cell_Temperatures : Outport  Port=4
  KnownSOC : Outport  Port=5  VectorParamsAs1DForOutWhenUnconnected=off
  wires:
  Data Type Conversion/1 -> Pack_Voltage/1
  Data Type Conversion4/1 -> Cell_Voltages/1
  Data Type Conversion2/1 -> Cell_Temperatures/1
  Data Type Conversion3/1 -> KnownSOC/1
  PS-Simulink Converter5/1 -> Data Type Conversion1/1
  PS-Simulink Converter3/1 -> Data Type Conversion/1
  Data Type Conversion1/1 -> Pack_Current/1
  ? -> Data Type Conversion4/1
  ? -> Bias/1
  Selector/1 -> Data Type Conversion3/1
  ? -> Selector/1
  Bias/1 -> Data Type Conversion2/1
  BalCmd/1 -> Simulink-PS Converter1/1
  connections:
  Voltage Sensor4/RConn1 -- PS-Simulink Converter3/LConn1
  PS-Simulink Converter5/LConn1 -- Current Sensor/RConn1
  +Batt/RConn1 -- Voltage Sensor4/LConn1 -- ModuleType2/LConn3
  Voltage Sensor4/RConn2 -- -Batt/RConn1 -- Current Sensor/RConn2
  Simulink-PS Converter1/RConn1 -- ModuleType2/LConn1
  Current Sensor/LConn1 -- ModuleType2/RConn1

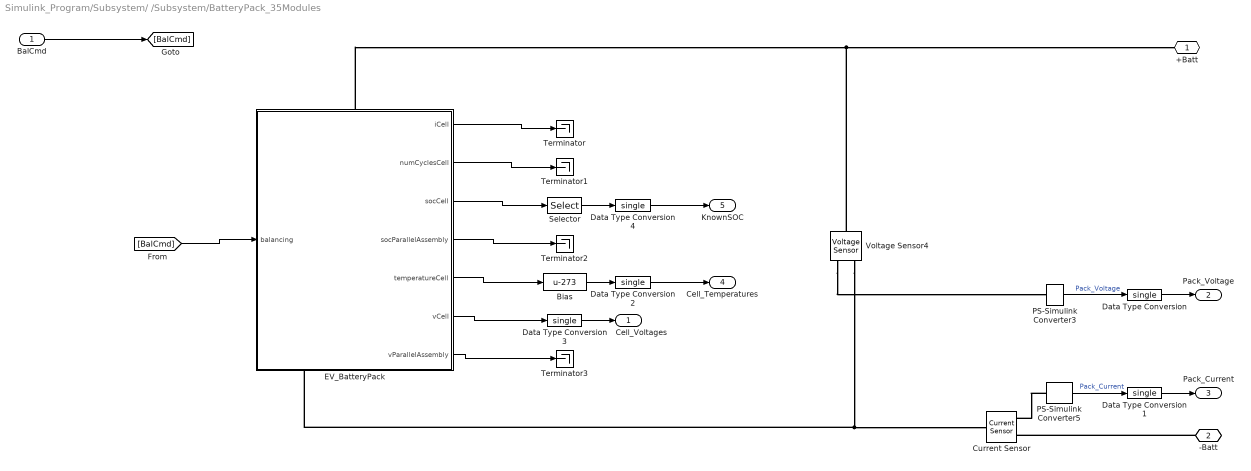
== system Simulink_Program/Subsystem/ /Subsystem/BatteryPack_35Modules ==
  BalCmd : Inport
  Bias : Bias  Bias=-273  SaturateOnIntegerOverflow=off
  Current Sensor : fl_lib/Electrical/Electrical Sensors/Current Sensor
  Data Type Conversion{,1..4} (5 alike) : DataTypeConversion  OutDataTypeStr=single  SaturateOnIntegerOverflow=off  RndMeth=Floor
  EV_BatteryPack : Subsystem  LoadFcn=battery_builder_rtmsupport('loadfcn',gcbh);
      settings: CopyFcn=battery_builder_rtmsupport('copyfcn',gcbh);  PreCopyFcn=battery_builder_rtmsupport('precopyfcn',gcbh);  PreDeleteFcn=battery_builder_rtmsupport('predeletefcn',gcbh);  PortSchema="{\"entries\":[{\"content\":{\"sides\":[{\"content\":{\"connectorIds\":[\"LConn1\"]},\"type\":\"ConnectorPlacement.EquallySpacedRectSide\",\"uuid\":\"65ed1d6a-8bbc-435f-b049-2af38d759a70\"},{\"content\":{\"connectorIds\":[\"RConn1\",\"RConn2\"],\"side\":\"RIGHT\"},\"type\":\"ConnectorPlacement.EquallySpacedRectSide\",\"uuid\":\"a1401bb9-5059-4839-a7a9-dd6fe2dda165\"},{\"content\":{\"connectorIds\":[\"In1\"],\"side\":\"TOP\"},\"type\":\"ConnectorPlacement.EquallySpacedRectSide\",\"uuid\":\"2c66cf8a-7c0d-404f-be4f-1afbd4c18bcf\"},{\"content\":{\"connectorIds\":[\"Out1\",\"Out2\",\"Out3\",\"Out4\",\"Out5\",\"Out6\",\"Out7\"],\"side\":\"BOTTOM\"},\"type\":\"ConnectorPlacement.EquallySpacedRectSide\",\"uuid\":\"a91736c9-9289-4be0-8d31-607fefcfa07a\"}]},\"type\":\"ConnectorPlacement.EquallySpacedConnector\",\"uuid\":\"29deba9c-4168-4045-8e33-2f9eda1ecc72\"}],\"packageUris\":[\"http://schema.mathworks.com/mf0/Connector/R2020b\"],\"version\":\"1.0\"}"
      mask Display: image('$imagefile')
  PS-Simulink Converter3 : nesl_utility/PS-Simulink Converter  PhysicalDomain=network_engine_domain  SubClassName=ps_output  LeftPortType=input  RightPortType=output  PseudoPeriodic=off  Frequencies=[]  VectorFormat=1-D array  Unit=V  AffineConversion=off
  PS-Simulink Converter5 : nesl_utility/PS-Simulink Converter  PhysicalDomain=network_engine_domain  SubClassName=ps_output  LeftPortType=input  RightPortType=output  PseudoPeriodic=off  Frequencies=[]  VectorFormat=1-D array  Unit=A  AffineConversion=off
  Selector : Selector  InputPortWidth=NumModules*Ns_Module  IndexOptions=Index vector (dialog)  Indices=1  OutputSizes=1
  Terminator{,1..3} (4 alike) : Terminator
  Voltage Sensor4 : fl_lib/Electrical/Electrical Sensors/Voltage Sensor
  +Batt : PMIOPort  Side=Right
  -Batt : PMIOPort  Port=2  Side=Right
  Cell_Voltages : Outport  VectorParamsAs1DForOutWhenUnconnected=off
  Pack_Voltage : Outport  Port=2  Unit=V  VectorParamsAs1DForOutWhenUnconnected=off
  Pack_Current : Outport  Port=3  Unit=A  VectorParamsAs1DForOutWhenUnconnected=off
  Cell_Temperatures : Outport  Port=4  VectorParamsAs1DForOutWhenUnconnected=off
  KnownSOC : Outport  Port=5
  wires:
  BalCmd/1 -> [BalCmd]
  PS-Simulink Converter3/1 -> Data Type Conversion/1  "Pack_Voltage"
  PS-Simulink Converter5/1 -> Data Type Conversion1/1  "Pack_Current"
  Data Type Conversion/1 -> Pack_Voltage/1
  Data Type Conversion1/1 -> Pack_Current/1
  Data Type Conversion2/1 -> Cell_Temperatures/1
  Data Type Conversion3/1 -> Cell_Voltages/1
  EV_BatteryPack/1(iCell) -> Terminator/1
  EV_BatteryPack/2(numCyclesCell) -> Terminator1/1
  EV_BatteryPack/3(socCell) -> Selector/1
  EV_BatteryPack/4(socParallelAssembly) -> Terminator2/1
  EV_BatteryPack/5(temperatureCell) -> Bias/1
  Bias/1 -> Data Type Conversion2/1
  EV_BatteryPack/6(vCell) -> Data Type Conversion3/1
  EV_BatteryPack/7(vParallelAssembly) -> Terminator3/1
  [BalCmd] -> EV_BatteryPack/1(balancing)
  Selector/1 -> Data Type Conversion4/1
  Data Type Conversion4/1 -> KnownSOC/1
  connections:
  -Batt/RConn1 -- Current Sensor/RConn2
  Voltage Sensor4/RConn1 -- PS-Simulink Converter3/LConn1
  PS-Simulink Converter5/LConn1 -- Current Sensor/RConn1
  Voltage Sensor4/LConn1 -- +Batt/RConn1 -- EV_BatteryPack/LConn1
  Voltage Sensor4/RConn2 -- Current Sensor/LConn1 -- EV_BatteryPack/RConn1

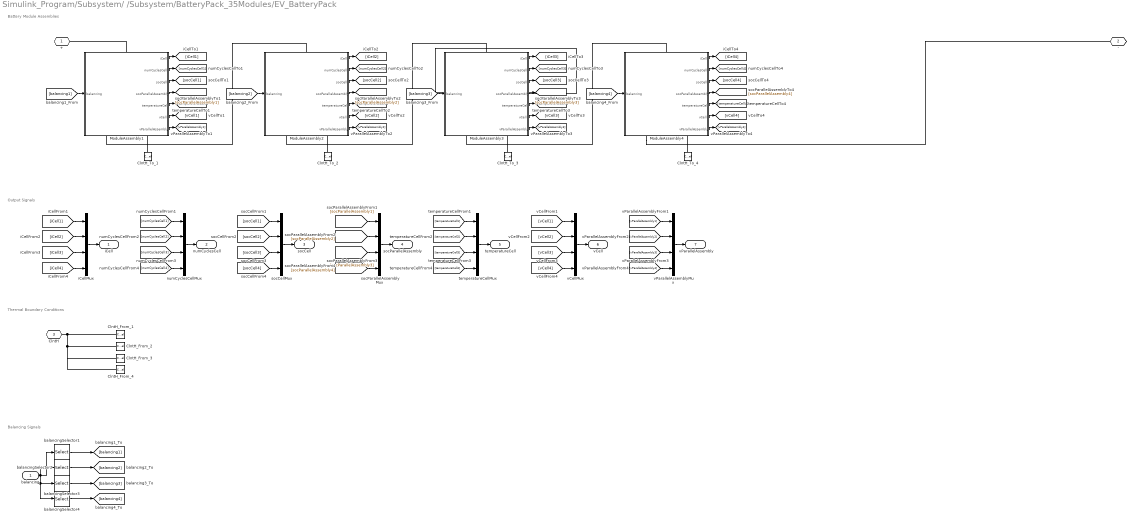
== system Simulink_Program/Subsystem/ /Subsystem/BatteryPack_35Modules/EV_BatteryPack ==
  note: Battery Module Assemblies
  note: Output Signals
  note: Thermal Boundary Conditions
  note: Balancing Signals
  balancing : Inport  PortDimensions=105
  ClntH_From_1 : ConnectionLabel  Label=clntH_1
  ClntH_From_2 : ConnectionLabel  Label=clntH_2
  ClntH_From_3 : ConnectionLabel  Label=clntH_3
  ClntH_From_4 : ConnectionLabel  Label=clntH_4
  ClntH_To_1 : ConnectionLabel  Label=clntH_1
  ClntH_To_2 : ConnectionLabel  Label=clntH_2
  ClntH_To_3 : ConnectionLabel  Label=clntH_3
  ClntH_To_4 : ConnectionLabel  Label=clntH_4
  ModuleAssembly1 : Subsystem  LoadFcn=battery_builder_rtmsupport('loadfcn',gcbh);
      settings: CopyFcn=battery_builder_rtmsupport('copyfcn',gcbh);  PreCopyFcn=battery_builder_rtmsupport('precopyfcn',gcbh);  PreDeleteFcn=battery_builder_rtmsupport('predeletefcn',gcbh);  PortSchema="{\"entries\":[{\"content\":{\"sides\":[{\"content\":{\"connectorIds\":[\"LConn1\"]},\"type\":\"ConnectorPlacement.EquallySpacedRectSide\",\"uuid\":\"65ed1d6a-8bbc-435f-b049-2af38d759a70\"},{\"content\":{\"connectorIds\":[\"RConn1\",\"RConn2\"],\"side\":\"RIGHT\"},\"type\":\"ConnectorPlacement.EquallySpacedRectSide\",\"uuid\":\"a1401bb9-5059-4839-a7a9-dd6fe2dda165\"},{\"content\":{\"connectorIds\":[\"In1\"],\"side\":\"TOP\"},\"type\":\"ConnectorPlacement.EquallySpacedRectSide\",\"uuid\":\"2c66cf8a-7c0d-404f-be4f-1afbd4c18bcf\"},{\"content\":{\"connectorIds\":[\"Out1\",\"Out2\",\"Out3\",\"Out4\",\"Out5\",\"Out6\",\"Out7\"],\"side\":\"BOTTOM\"},\"type\":\"ConnectorPlacement.EquallySpacedRectSide\",\"uuid\":\"b1a645e2-0220-4984-a761-2404f3742cb8\"}]},\"type\":\"ConnectorPlacement.EquallySpacedConnector\",\"uuid\":\"29deba9c-4168-4045-8e33-2f9eda1ecc72\"}],\"packageUris\":[\"http://schema.mathworks.com/mf0/Connector/R2020b\"],\"version\":\"1.0\"}"
      mask Display: image('$imagefile')
  ModuleAssembly2 : Subsystem  LoadFcn=battery_builder_rtmsupport('loadfcn',gcbh);
      settings: CopyFcn=battery_builder_rtmsupport('copyfcn',gcbh);  PreCopyFcn=battery_builder_rtmsupport('precopyfcn',gcbh);  PreDeleteFcn=battery_builder_rtmsupport('predeletefcn',gcbh);  PortSchema="{\"entries\":[{\"content\":{\"sides\":[{\"content\":{\"connectorIds\":[\"LConn1\"]},\"type\":\"ConnectorPlacement.EquallySpacedRectSide\",\"uuid\":\"65ed1d6a-8bbc-435f-b049-2af38d759a70\"},{\"content\":{\"connectorIds\":[\"RConn1\",\"RConn2\"],\"side\":\"RIGHT\"},\"type\":\"ConnectorPlacement.EquallySpacedRectSide\",\"uuid\":\"a1401bb9-5059-4839-a7a9-dd6fe2dda165\"},{\"content\":{\"connectorIds\":[\"In1\"],\"side\":\"TOP\"},\"type\":\"ConnectorPlacement.EquallySpacedRectSide\",\"uuid\":\"2c66cf8a-7c0d-404f-be4f-1afbd4c18bcf\"},{\"content\":{\"connectorIds\":[\"Out1\",\"Out2\",\"Out3\",\"Out4\",\"Out5\",\"Out6\",\"Out7\"],\"side\":\"BOTTOM\"},\"type\":\"ConnectorPlacement.EquallySpacedRectSide\",\"uuid\":\"b1a645e2-0220-4984-a761-2404f3742cb8\"}]},\"type\":\"ConnectorPlacement.EquallySpacedConnector\",\"uuid\":\"29deba9c-4168-4045-8e33-2f9eda1ecc72\"}],\"packageUris\":[\"http://schema.mathworks.com/mf0/Connector/R2020b\"],\"version\":\"1.0\"}"
      mask Display: image('$imagefile')
  ModuleAssembly3 : Subsystem  LoadFcn=battery_builder_rtmsupport('loadfcn',gcbh);
      settings: CopyFcn=battery_builder_rtmsupport('copyfcn',gcbh);  PreCopyFcn=battery_builder_rtmsupport('precopyfcn',gcbh);  PreDeleteFcn=battery_builder_rtmsupport('predeletefcn',gcbh);  PortSchema="{\"entries\":[{\"content\":{\"sides\":[{\"content\":{\"connectorIds\":[\"LConn1\"]},\"type\":\"ConnectorPlacement.EquallySpacedRectSide\",\"uuid\":\"65ed1d6a-8bbc-435f-b049-2af38d759a70\"},{\"content\":{\"connectorIds\":[\"RConn1\",\"RConn2\"],\"side\":\"RIGHT\"},\"type\":\"ConnectorPlacement.EquallySpacedRectSide\",\"uuid\":\"a1401bb9-5059-4839-a7a9-dd6fe2dda165\"},{\"content\":{\"connectorIds\":[\"In1\"],\"side\":\"TOP\"},\"type\":\"ConnectorPlacement.EquallySpacedRectSide\",\"uuid\":\"2c66cf8a-7c0d-404f-be4f-1afbd4c18bcf\"},{\"content\":{\"connectorIds\":[\"Out1\",\"Out2\",\"Out3\",\"Out4\",\"Out5\",\"Out6\",\"Out7\"],\"side\":\"BOTTOM\"},\"type\":\"ConnectorPlacement.EquallySpacedRectSide\",\"uuid\":\"b1a645e2-0220-4984-a761-2404f3742cb8\"}]},\"type\":\"ConnectorPlacement.EquallySpacedConnector\",\"uuid\":\"29deba9c-4168-4045-8e33-2f9eda1ecc72\"}],\"packageUris\":[\"http://schema.mathworks.com/mf0/Connector/R2020b\"],\"version\":\"1.0\"}"
      mask Display: image('$imagefile')
  ModuleAssembly4 : Subsystem  LoadFcn=battery_builder_rtmsupport('loadfcn',gcbh);
      settings: CopyFcn=battery_builder_rtmsupport('copyfcn',gcbh);  PreCopyFcn=battery_builder_rtmsupport('precopyfcn',gcbh);  PreDeleteFcn=battery_builder_rtmsupport('predeletefcn',gcbh);  PortSchema="{\"entries\":[{\"content\":{\"sides\":[{\"content\":{\"connectorIds\":[\"LConn1\"]},\"type\":\"ConnectorPlacement.EquallySpacedRectSide\",\"uuid\":\"65ed1d6a-8bbc-435f-b049-2af38d759a70\"},{\"content\":{\"connectorIds\":[\"RConn1\",\"RConn2\"],\"side\":\"RIGHT\"},\"type\":\"ConnectorPlacement.EquallySpacedRectSide\",\"uuid\":\"a1401bb9-5059-4839-a7a9-dd6fe2dda165\"},{\"content\":{\"connectorIds\":[\"In1\"],\"side\":\"TOP\"},\"type\":\"ConnectorPlacement.EquallySpacedRectSide\",\"uuid\":\"2c66cf8a-7c0d-404f-be4f-1afbd4c18bcf\"},{\"content\":{\"connectorIds\":[\"Out1\",\"Out2\",\"Out3\",\"Out4\",\"Out5\",\"Out6\",\"Out7\"],\"side\":\"BOTTOM\"},\"type\":\"ConnectorPlacement.EquallySpacedRectSide\",\"uuid\":\"7f78025c-dd25-4844-b041-d03b271c9ab1\"}]},\"type\":\"ConnectorPlacement.EquallySpacedConnector\",\"uuid\":\"29deba9c-4168-4045-8e33-2f9eda1ecc72\"}],\"packageUris\":[\"http://schema.mathworks.com/mf0/Connector/R2020b\"],\"version\":\"1.0\"}"
      mask Display: image('$imagefile')
  balancingSelector1 : Selector  InputPortWidth=105  IndexOptions=Index vector (dialog)  Indices="[1   2   3   4   5   6   7   8   9  10  11  12  13  14  15  16  17  18  19  20  21  22  23  24  25  26  27]"  OutputSizes=1
  balancingSelector2 : Selector  InputPortWidth=105  IndexOptions=Index vector (dialog)  Indices="[28  29  30  31  32  33  34  35  36  37  38  39  40  41  42  43  44  45  46  47  48  49  50  51  52  53  54]"  OutputSizes=1
  balancingSelector3 : Selector  InputPortWidth=105  IndexOptions=Index vector (dialog)  Indices="[55  56  57  58  59  60  61  62  63  64  65  66  67  68  69  70  71  72  73  74  75  76  77  78  79  80  81]"  OutputSizes=1
  balancingSelector4 : Selector  InputPortWidth=105  IndexOptions=Index vector (dialog)  Indices="[82   83   84   85   86   87   88   89   90   91   92   93   94   95   96   97   98   99  100  101  102  103  104  105]"  OutputSizes=1
  iCellMux : Mux
  numCyclesCellMux : Mux
  socCellMux : Mux
  socParallelAssemblyMux : Mux
  temperatureCellMux : Mux
  vCellMux : Mux
  vParallelAssemblyMux : Mux
  + : PMIOPort  Side=Left
  - : PMIOPort  Port=2  Side=Right
  ClntH : PMIOPort  Port=3  Side=Right  ConnectionType=Connection: foundation.thermal.thermal
  iCell : Outport
  numCyclesCell : Outport  Port=2
  socCell : Outport  Port=3
  socParallelAssembly : Outport  Port=4
  temperatureCell : Outport  Port=5
  vCell : Outport  Port=6
  vParallelAssembly : Outport  Port=7
  wires:
  ModuleAssembly1/1(iCell) -> [iCell1]
  iCellMux/1 -> iCell/1
  [iCell1] -> iCellMux/1
  ModuleAssembly1/2(numCyclesCell) -> [numCyclesCell1]
  numCyclesCellMux/1 -> numCyclesCell/1
  [numCyclesCell1] -> numCyclesCellMux/1
  ModuleAssembly1/3(socCell) -> [socCell1]
  socCellMux/1 -> socCell/1
  [socCell1] -> socCellMux/1
  ModuleAssembly1/4(socParallelAssembly) -> [socParallelAssembly1]
  socParallelAssemblyMux/1 -> socParallelAssembly/1
  [socParallelAssembly1] -> socParallelAssemblyMux/1
  ModuleAssembly1/5(temperatureCell) -> [temperatureCell1]
  temperatureCellMux/1 -> temperatureCell/1
  [temperatureCell1] -> temperatureCellMux/1
  ModuleAssembly1/6(vCell) -> [vCell1]
  vCellMux/1 -> vCell/1
  [vCell1] -> vCellMux/1
  ModuleAssembly1/7(vParallelAssembly) -> [vParallelAssembly1]
  vParallelAssemblyMux/1 -> vParallelAssembly/1
  [vParallelAssembly1] -> vParallelAssemblyMux/1
  ModuleAssembly2/1(iCell) -> [iCell2]
  [iCell2] -> iCellMux/2
  ModuleAssembly2/2(numCyclesCell) -> [numCyclesCell2]
  [numCyclesCell2] -> numCyclesCellMux/2
  ModuleAssembly2/3(socCell) -> [socCell2]
  [socCell2] -> socCellMux/2
  ModuleAssembly2/4(socParallelAssembly) -> [socParallelAssembly2]
  [socParallelAssembly2] -> socParallelAssemblyMux/2
  ModuleAssembly2/5(temperatureCell) -> [temperatureCell2]
  [temperatureCell2] -> temperatureCellMux/2
  ModuleAssembly2/6(vCell) -> [vCell2]
  [vCell2] -> vCellMux/2
  ModuleAssembly2/7(vParallelAssembly) -> [vParallelAssembly2]
  [vParallelAssembly2] -> vParallelAssemblyMux/2
  ModuleAssembly3/1(iCell) -> [iCell3]
  [iCell3] -> iCellMux/3
  ModuleAssembly3/2(numCyclesCell) -> [numCyclesCell3]
  [numCyclesCell3] -> numCyclesCellMux/3
  ModuleAssembly3/3(socCell) -> [socCell3]
  [socCell3] -> socCellMux/3
  ModuleAssembly3/4(socParallelAssembly) -> [socParallelAssembly3]
  [socParallelAssembly3] -> socParallelAssemblyMux/3
  ModuleAssembly3/5(temperatureCell) -> [temperatureCell3]
  [temperatureCell3] -> temperatureCellMux/3
  ModuleAssembly3/6(vCell) -> [vCell3]
  [vCell3] -> vCellMux/3
  ModuleAssembly3/7(vParallelAssembly) -> [vParallelAssembly3]
  [vParallelAssembly3] -> vParallelAssemblyMux/3
  ModuleAssembly4/1(iCell) -> [iCell4]
  [iCell4] -> iCellMux/4
  ModuleAssembly4/2(numCyclesCell) -> [numCyclesCell4]
  [numCyclesCell4] -> numCyclesCellMux/4
  ModuleAssembly4/3(socCell) -> [socCell4]
  [socCell4] -> socCellMux/4
  ModuleAssembly4/4(socParallelAssembly) -> [socParallelAssembly4]
  [socParallelAssembly4] -> socParallelAssemblyMux/4
  ModuleAssembly4/5(temperatureCell) -> [temperatureCell4]
  [temperatureCell4] -> temperatureCellMux/4
  ModuleAssembly4/6(vCell) -> [vCell4]
  [vCell4] -> vCellMux/4
  ModuleAssembly4/7(vParallelAssembly) -> [vParallelAssembly4]
  [vParallelAssembly4] -> vParallelAssemblyMux/4
  [balancing1] -> ModuleAssembly1/1(balancing)
  balancing/1 -> balancingSelector3/1, balancingSelector4/1, balancingSelector1/1, balancingSelector2/1
  balancingSelector1/1 -> [balancing1]
  [balancing2] -> ModuleAssembly2/1(balancing)
  balancingSelector2/1 -> [balancing2]
  [balancing3] -> ModuleAssembly3/1(balancing)
  balancingSelector3/1 -> [balancing3]
  [balancing4] -> ModuleAssembly4/1(balancing)
  balancingSelector4/1 -> [balancing4]
  connections:
  ModuleAssembly2/LConn1 -- ModuleAssembly1/RConn1
  ModuleAssembly3/LConn1 -- ModuleAssembly2/RConn1
  ModuleAssembly4/LConn1 -- ModuleAssembly3/RConn1
  ModuleAssembly1/LConn1 -- +/RConn1
  ModuleAssembly4/RConn1 -- -/RConn1
  ClntH_To_1/LConn1 -- ModuleAssembly1/RConn2
  ClntH/RConn1 -- ClntH_From_1/LConn1 -- ClntH_From_2/LConn1 -- ClntH_From_4/LConn1 -- ClntH_From_3/LConn1
  ClntH_To_2/LConn1 -- ModuleAssembly2/RConn2
  ClntH_To_3/LConn1 -- ModuleAssembly3/RConn2
  ClntH_To_4/LConn1 -- ModuleAssembly4/RConn2
